simulink model "mrefrobotarm_modified_previous_y_previous_u_previous_ref_prepro"  (R2018b)
settings: Solver=FixedStepAuto  StartTime=0.0  StopTime=10  RelTol=1e-3  AbsTol=1e-6
undefined symbols (not defined in the file or in its folder): cc, options
libraries: neural x594, simulink x1
(part 4 of 22)

== system mrefrobotarm_modified_previous_y_previous_u_previous_ref_prepro/pre_0.01/Layer 3 ==
  "a{2} " : Inport  PortDimensions=30
      mask Display: e = 0.06;c1 = [120 230 180]/255;c2 = ([120 230 180]+0)/(256+128);c3 = ([120 230 180]+128)/(256+128);patch([0 1 1 0],[0 0 1 1],c1);patch([0 1 1 1-e 1-e 0+e],[0 0 1 1-e 0+e 0+e],c2);patch([0 0 1 1-e 0+e 0+e],[0 1 1 1-e 1-e 0+e],c3);plot([0 1 1 0 0],[0 0 1 1 0]);
  Delays 1 : Subsystem
      mask Display: e = 0.06;c1 = [120 150 230]/255;c2 = ([120 150 230]+0)/383;c3 = ([120 150 230]+128)/383;patch([0 1 1 0],[0 0 1 1],c1);patch([0 1 1 1-e 1-e 0+e],[0 0 1 1-e 0+e 0+e],c2);patch([0 0 1 1-e 0+e 0+e],[0 1 1 1-e 1-e 0+e],c3);plot([0 1 1 0 0],[0 0 1 1 0]);disp('0');
  "LW{3,2}" : Subsystem
      mask Display: e = 0.06;c1 = [120 150 230]/255;c2 = ([120 150 230]+0)/383;c3 = ([120 150 230]+128)/383;patch([0 1 1 0],[0 0 1 1],c1);patch([0 1 1 1-e 1-e 0+e],[0 0 1 1-e 0+e 0+e],c2);patch([0 0 1 1-e 0+e 0+e],[0 1 1 1-e 1-e 0+e],c3);plot([0 1 1 0 0],[0 0 1 1 0]);disp('W');
  "b{3}" : Constant  Value=0.10618203195990393028491638460764079354703426361083984375
      mask Display: e = 0.06;c1 = [120 150 230]/255;c2 = ([120 150 230]+0)/383;c3 = ([120 150 230]+128)/383;patch([0 1 1 0],[0 0 1 1],c1);patch([0 1 1 1-e 1-e 0+e],[0 0 1 1-e 0+e 0+e],c2);patch([0 0 1 1-e 0+e 0+e],[0 1 1 1-e 1-e 0+e],c3);plot([0 1 1 0 0],[0 0 1 1 0]);disp('b');
  netsum : Sum  Inputs=2  SaturateOnIntegerOverflow=on  InputSameDT=on  OutDataTypeStr=Inherit: Same as first input
      mask Display: e = 0.06;c1 = [120 150 230]/255;c2 = ([120 150 230]+0)/383;c3 = ([120 150 230]+128)/383;patch([0 1 1 0],[0 0 1 1],c1);patch([0 1 1 1-e 1-e 0+e],[0 0 1 1-e 0+e 0+e],c2);patch([0 0 1 1-e 0+e 0+e],[0 1 1 1-e 1-e 0+e],c3);plot([0 1 1 0 0],[0 0 1 1 0]);disp('+');
  purelin : neural/Transfer Functions/purelin
  "a{3}" : Outport  InitialOutput=0
      mask Display: e = 0.06;c1 = [120 230 180]/255;c2 = ([120 230 180]+0)/(256+128);c3 = ([120 230 180]+128)/(256+128);patch([0 1 1 0],[0 0 1 1],c1);patch([0 1 1 1-e 1-e 0+e],[0 0 1 1-e 0+e 0+e],c2);patch([0 0 1 1-e 0+e 0+e],[0 1 1 1-e 1-e 0+e],c3);plot([0 1 1 0 0],[0 0 1 1 0]);
  wires:
  "a{2} "/1 -> Delays 1/1("p{3}")
  Delays 1/1("pd{3,2}") -> "LW{3,2}"/1("ad{3,2}")
  "LW{3,2}"/1("lz{3,2}") -> netsum/1
  "b{3}"/1 -> netsum/2
  netsum/1 -> purelin/1
  purelin/1 -> "a{3}"/1

== system mrefrobotarm_modified_previous_y_previous_u_previous_ref_prepro/pre_0.01/Process Input 1 ==
  x : Inport  PortDimensions=10
      mask Display: e = 0.06;c1 = [120 230 180]/255;c2 = ([120 230 180]+0)/(256+128);c3 = ([120 230 180]+128)/(256+128);patch([0 1 1 0],[0 0 1 1],c1);patch([0 1 1 1-e 1-e 0+e],[0 0 1 1-e 0+e 0+e],c2);patch([0 0 1 1-e 0+e 0+e],[0 1 1 1-e 1-e 0+e],c3);plot([0 1 1 0 0],[0 0 1 1 0]);
  mapminmax : neural/Processing Functions/mapminmax  xmin=[-0.499622681643638155701836467415;-0.499622681643638155701836467415;-0.499622681643638155701836467415;-0.499622681643638155701836467415;-0.521390823259639368814077897696;-0.521390823259639368814077897696;-0.521390823259639368814077897696;-0.521390823259639368814077897696;-181.831597500088662400230532512;-181.831597500088662400230532512]  xmax=[0.499081940855403360934872125654;0.499081940855403360934872125654;0.499081940855403360934872125654;0.499081940855403360934872125654;0.529053256590264919800858933741;0.529053256590264919800858933741;0.529053256590264919800858933741;0.529053256590264919800858933741;187.244110317709044011280639097;187.244110317709044011280639097]  ymin=-1  ymax=1
  p : Outport  PortDimensions=10
      mask Display: e = 0.06;c1 = [120 230 180]/255;c2 = ([120 230 180]+0)/(256+128);c3 = ([120 230 180]+128)/(256+128);patch([0 1 1 0],[0 0 1 1],c1);patch([0 1 1 1-e 1-e 0+e],[0 0 1 1-e 0+e 0+e],c2);patch([0 0 1 1-e 0+e 0+e],[0 1 1 1-e 1-e 0+e],c3);plot([0 1 1 0 0],[0 0 1 1 0]);
  wires:
  x/1 -> mapminmax/1
  mapminmax/1 -> p/1

== system mrefrobotarm_modified_previous_y_previous_u_previous_ref_prepro/pre_0.01/Process Output 1 ==
  a : Inport  PortDimensions=1
      mask Display: e = 0.06;c1 = [120 230 180]/255;c2 = ([120 230 180]+0)/(256+128);c3 = ([120 230 180]+128)/(256+128);patch([0 1 1 0],[0 0 1 1],c1);patch([0 1 1 1-e 1-e 0+e],[0 0 1 1-e 0+e 0+e],c2);patch([0 0 1 1-e 0+e 0+e],[0 1 1 1-e 1-e 0+e],c3);plot([0 1 1 0 0],[0 0 1 1 0]);
  mapminmax_reverse : neural/Processing Functions/mapminmax_reverse  xmin=-181.831597500088662400230532512  xmax=187.244110317709044011280639097  ymin=-1  ymax=1
  y : Outport  PortDimensions=1
      mask Display: e = 0.06;c1 = [120 230 180]/255;c2 = ([120 230 180]+0)/(256+128);c3 = ([120 230 180]+128)/(256+128);patch([0 1 1 0],[0 0 1 1],c1);patch([0 1 1 1-e 1-e 0+e],[0 0 1 1-e 0+e 0+e],c2);patch([0 0 1 1-e 0+e 0+e],[0 1 1 1-e 1-e 0+e],c3);plot([0 1 1 0 0],[0 0 1 1 0]);
  wires:
  a/1 -> mapminmax_reverse/1
  mapminmax_reverse/1 -> y/1

== system mrefrobotarm_modified_previous_y_previous_u_previous_ref_prepro/m=0.01 sd =0.01/Layer 1/Delays 1 ==
  "p{1}" : Inport  PortDimensions=10
      mask Display: e = 0.06;c1 = [120 230 180]/255;c2 = ([120 230 180]+0)/(256+128);c3 = ([120 230 180]+128)/(256+128);patch([0 1 1 0],[0 0 1 1],c1);patch([0 1 1 1-e 1-e 0+e],[0 0 1 1-e 0+e 0+e],c2);patch([0 0 1 1-e 0+e 0+e],[0 1 1 1-e 1-e 0+e],c3);plot([0 1 1 0 0],[0 0 1 1 0]);
  mux : Mux  Inputs=1
      mask Display: e = 0.06;c1 = [120 150 230]/255;c2 = ([120 150 230]+0)/383;c3 = ([120 150 230]+128)/383;patch([0 1 1 0],[0 0 1 1],c1);patch([0 1 1 1-e 1-e 0+e],[0 0 1 1-e 0+e 0+e],c2);patch([0 0 1 1-e 0+e 0+e],[0 1 1 1-e 1-e 0+e],c3);plot([0 1 1 0 0],[0 0 1 1 0]);disp('Mux')
  "pd{1,1}" : Outport
      mask Display: e = 0.06;c1 = [120 230 180]/255;c2 = ([120 230 180]+0)/(256+128);c3 = ([120 230 180]+128)/(256+128);patch([0 1 1 0],[0 0 1 1],c1);patch([0 1 1 1-e 1-e 0+e],[0 0 1 1-e 0+e 0+e],c2);patch([0 0 1 1-e 0+e 0+e],[0 1 1 1-e 1-e 0+e],c3);plot([0 1 1 0 0],[0 0 1 1 0]);
  wires:
  "p{1}"/1 -> mux/1
  mux/1 -> "pd{1,1}"/1

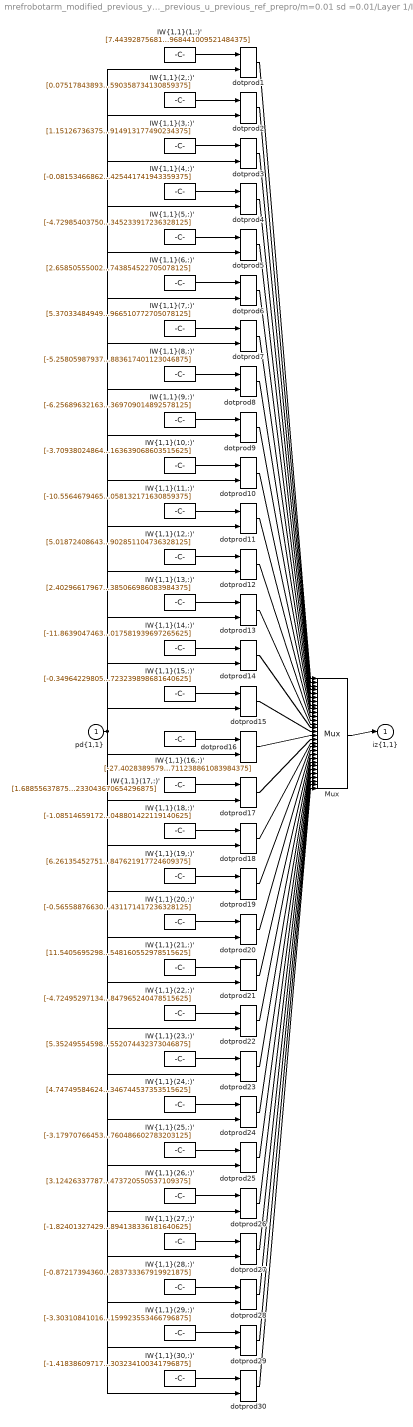
== system mrefrobotarm_modified_previous_y_previous_u_previous_ref_prepro/m=0.01 sd =0.01/Layer 1/IW{1,1} ==
  "pd{1,1}" : Inport  PortDimensions=10
      mask Display: e = 0.06;c1 = [120 230 180]/255;c2 = ([120 230 180]+0)/(256+128);c3 = ([120 230 180]+128)/(256+128);patch([0 1 1 0],[0 0 1 1],c1);patch([0 1 1 1-e 1-e 0+e],[0 0 1 1-e 0+e 0+e],c2);patch([0 0 1 1-e 0+e 0+e],[0 1 1 1-e 1-e 0+e],c3);plot([0 1 1 0 0],[0 0 1 1 0]);
  "IW{1,1}(1,:)'" : Constant  Value=[7.44392875681690302513970891595818102359771728515625;-4.6736656727683101308912227977998554706573486328125;-4.6390972498699891701789965736679732799530029296875;3.336024804118176145806273780181072652339935302734375;-0.105740361348570510724442783612175844609737396240234375;-3.024615511833397274443768765195272862911224365234375;2.36822163920083728072540907305665314197540283203125;-1.0457591878507825899902172750444151461124420166015625;1.046465722409650300761541075189597904682159423828125;-1.08392310721119056182715212344191968441009521484375]
      mask Display: e = 0.06;c1 = [120 150 230]/255;c2 = ([120 150 230]+0)/383;c3 = ([120 150 230]+128)/383;patch([0 1 1 0],[0 0 1 1],c1);patch([0 1 1 1-e 1-e 0+e],[0 0 1 1-e 0+e 0+e],c2);patch([0 0 1 1-e 0+e 0+e],[0 1 1 1-e 1-e 0+e],c3);plot([0 1 1 0 0],[0 0 1 1 0]);disp('Weights');
  "IW{1,1}(10,:)'" : Constant  Value=[-3.70938024864611026742977628600783646106719970703125;7.378455816069614314756108797155320644378662109375;-1.23455737014168942522474026191048324108123779296875;-0.80686346190143953815976374244200997054576873779296875;-2.678462781440510642738672686391510069370269775390625;-0.64571835168026459061962896157638169825077056884765625;0.99308648301582724826630510506220161914825439453125;0.0755819949909401211929349528872990049421787261962890625;-1.49364463106134603975760910543613135814666748046875;-1.0017750393580355794398428770364262163639068603515625]
      mask Display: e = 0.06;c1 = [120 150 230]/255;c2 = ([120 150 230]+0)/383;c3 = ([120 150 230]+128)/383;patch([0 1 1 0],[0 0 1 1],c1);patch([0 1 1 1-e 1-e 0+e],[0 0 1 1-e 0+e 0+e],c2);patch([0 0 1 1-e 0+e 0+e],[0 1 1 1-e 1-e 0+e],c3);plot([0 1 1 0 0],[0 0 1 1 0]);disp('Weights');
  "IW{1,1}(11,:)'" : Constant  Value=[-10.556467946534542790004707057960331439971923828125;5.98135936748858565437103607109747827053070068359375;3.653943008658041780023495448403991758823394775390625;-0.11845730388351143058667247487392160110175609588623046875;0.3526287060857471455932454773574136197566986083984375;1.7762225366593791253677636632346548140048980712890625;-1.37767047732931313674953344161622226238250732421875;-0.63824863500093720336536762260948307812213897705078125;0.8549609373443776139112060263869352638721466064453125;0.642023567932097360966281485161744058132171630859375]
      mask Display: e = 0.06;c1 = [120 150 230]/255;c2 = ([120 150 230]+0)/383;c3 = ([120 150 230]+128)/383;patch([0 1 1 0],[0 0 1 1],c1);patch([0 1 1 1-e 1-e 0+e],[0 0 1 1-e 0+e 0+e],c2);patch([0 0 1 1-e 0+e 0+e],[0 1 1 1-e 1-e 0+e],c3);plot([0 1 1 0 0],[0 0 1 1 0]);disp('Weights');
  "IW{1,1}(12,:)'" : Constant  Value=[5.018724086434847464488484547473490238189697265625;-4.47618638864089124496103977435268461704254150390625;1.4027950886756685999756655292003415524959564208984375;-0.01760069917661223615201748771141865290701389312744140625;0.06580408721141249583919119459096691571176052093505859375;-0.435612092762941827128742033892194740474224090576171875;-0.123377444074154851705316104926168918609619140625;1.513619026736596762106046298868022859096527099609375;-0.2081431014525624567657047236934886313974857330322265625;0.72520741288983459060801806117524392902851104736328125]
      mask Display: e = 0.06;c1 = [120 150 230]/255;c2 = ([120 150 230]+0)/383;c3 = ([120 150 230]+128)/383;patch([0 1 1 0],[0 0 1 1],c1);patch([0 1 1 1-e 1-e 0+e],[0 0 1 1-e 0+e 0+e],c2);patch([0 0 1 1-e 0+e 0+e],[0 1 1 1-e 1-e 0+e],c3);plot([0 1 1 0 0],[0 0 1 1 0]);disp('Weights');
  "IW{1,1}(13,:)'" : Constant  Value=[2.402966179675783298108626695466227829456329345703125;-1.6093946888288417351731141025084070861339569091796875;-0.0599342394857917681871839477025787346065044403076171875;-0.473275413721871374139738009034772403538227081298828125;-0.87682561446088513879004722184618003666400909423828125;0.22628827655378025429655508560244925320148468017578125;0.444344236189617103338633796738577075302600860595703125;-0.329101618948661689412205078042461536824703216552734375;-0.74224906653537059408876075394800864160060882568359375;-0.198310173910472453684405991225503385066986083984375]
      mask Display: e = 0.06;c1 = [120 150 230]/255;c2 = ([120 150 230]+0)/383;c3 = ([120 150 230]+128)/383;patch([0 1 1 0],[0 0 1 1],c1);patch([0 1 1 1-e 1-e 0+e],[0 0 1 1-e 0+e 0+e],c2);patch([0 0 1 1-e 0+e 0+e],[0 1 1 1-e 1-e 0+e],c3);plot([0 1 1 0 0],[0 0 1 1 0]);disp('Weights');
  "IW{1,1}(14,:)'" : Constant  Value=[-11.863904746364600129027166985906660556793212890625;12.5361553086397687906128339818678796291351318359375;-2.5443094142737994189928940613754093647003173828125;-0.01039113964185867967915388732080828049220144748687744140625;-1.4967394616593383549485452022054232656955718994140625;2.8221017636860725730230115004815161228179931640625;-0.1929962862818650481955273789935745298862457275390625;-2.793854429713266807056015750276856124401092529296875;-0.55739373934864355764062793241464532911777496337890625;-1.942644023618106619011314251110889017581939697265625]
      mask Display: e = 0.06;c1 = [120 150 230]/255;c2 = ([120 150 230]+0)/383;c3 = ([120 150 230]+128)/383;patch([0 1 1 0],[0 0 1 1],c1);patch([0 1 1 1-e 1-e 0+e],[0 0 1 1-e 0+e 0+e],c2);patch([0 0 1 1-e 0+e 0+e],[0 1 1 1-e 1-e 0+e],c3);plot([0 1 1 0 0],[0 0 1 1 0]);disp('Weights');
  "IW{1,1}(15,:)'" : Constant  Value=[-0.349642298058042089170527333408244885504245758056640625;2.606095277319749659028502719593234360218048095703125;-1.2963224095569134686201095973956398665904998779296875;-1.6246252820403725980469289424945600330829620361328125;4.39476319833291118044371614814735949039459228515625;0.327169101324004507613807390953297726809978485107421875;-3.431185950754114255545346168219111859798431396484375;0.82290277565416491967198453494347631931304931640625;1.922123395477147056453759432770311832427978515625;1.617192821484084053196284003206528723239898681640625]
      mask Display: e = 0.06;c1 = [120 150 230]/255;c2 = ([120 150 230]+0)/383;c3 = ([120 150 230]+128)/383;patch([0 1 1 0],[0 0 1 1],c1);patch([0 1 1 1-e 1-e 0+e],[0 0 1 1-e 0+e 0+e],c2);patch([0 0 1 1-e 0+e 0+e],[0 1 1 1-e 1-e 0+e],c3);plot([0 1 1 0 0],[0 0 1 1 0]);disp('Weights');
  "IW{1,1}(16,:)'" : Constant  Value=[-27.402838957925386154101943247951567173004150390625;27.31809732638254217818030156195163726806640625;4.187796846523848870447181980125606060028076171875;-0.58411520480238465768962896618177182972431182861328125;-2.421077128426197599964098117197863757610321044921875;-0.422057029001945249735427978521329350769519805908203125;0.46933164629719448246447655037627555429935455322265625;2.53884227966835052114902282482944428920745849609375;0.449642930046671496224774955408065579831600189208984375;-1.6588674943129804173480579265742562711238861083984375]
      mask Display: e = 0.06;c1 = [120 150 230]/255;c2 = ([120 150 230]+0)/383;c3 = ([120 150 230]+128)/383;patch([0 1 1 0],[0 0 1 1],c1);patch([0 1 1 1-e 1-e 0+e],[0 0 1 1-e 0+e 0+e],c2);patch([0 0 1 1-e 0+e 0+e],[0 1 1 1-e 1-e 0+e],c3);plot([0 1 1 0 0],[0 0 1 1 0]);disp('Weights');
  "IW{1,1}(17,:)'" : Constant  Value=[1.6885563787544148883768002633587457239627838134765625;-2.444624938858031004684789877501316368579864501953125;1.2252322902321706177275473237386904656887054443359375;-0.590265120460011782910214606090448796749114990234375;-0.332311297209722800172215784186846576631069183349609375;0.96575580482126255343899856598000042140483856201171875;-0.00354470077974646143037507073358938214369118213653564453125;-0.1126520435161915412169975070355576463043689727783203125;-0.33787689238072371455956499630701728165149688720703125;0.82478955221782601636704157499480061233043670654296875]
      mask Display: e = 0.06;c1 = [120 150 230]/255;c2 = ([120 150 230]+0)/383;c3 = ([120 150 230]+128)/383;patch([0 1 1 0],[0 0 1 1],c1);patch([0 1 1 1-e 1-e 0+e],[0 0 1 1-e 0+e 0+e],c2);patch([0 0 1 1-e 0+e 0+e],[0 1 1 1-e 1-e 0+e],c3);plot([0 1 1 0 0],[0 0 1 1 0]);disp('Weights');
  "IW{1,1}(18,:)'" : Constant  Value=[-1.0851465917204592415146180428564548492431640625;2.2300343259938220086269211606122553348541259765625;-0.275391438559908163785650003774208016693592071533203125;-0.3928571879931632704341382122947834432125091552734375;0.354493692437090335278782049499568529427051544189453125;-0.420219301105624498671176070274668745696544647216796875;-0.11256805056305159429275164484351989813148975372314453125;0.133925253068311878035245854334789328277111053466796875;-0.319742826625007747765039312071166932582855224609375;0.1931074981940363033405816395315923728048801422119140625]
      mask Display: e = 0.06;c1 = [120 150 230]/255;c2 = ([120 150 230]+0)/383;c3 = ([120 150 230]+128)/383;patch([0 1 1 0],[0 0 1 1],c1);patch([0 1 1 1-e 1-e 0+e],[0 0 1 1-e 0+e 0+e],c2);patch([0 0 1 1-e 0+e 0+e],[0 1 1 1-e 1-e 0+e],c3);plot([0 1 1 0 0],[0 0 1 1 0]);disp('Weights');
  "IW{1,1}(19,:)'" : Constant  Value=[6.2613545275196411665774576249532401561737060546875;-5.77393711359606864874649545527063310146331787109375;-0.44799036385010515548543708064244128763675689697265625;0.13038042920451109463186867287731729447841644287109375;-1.1128052994417583221320455777458846569061279296875;-0.68497464755320169871311009046621620655059814453125;1.488082305967609375585425368626601994037628173828125;-0.58498852802415501894728322440641932189464569091796875;-0.72696347840742070456343526529963128268718719482421875;-0.91570155227344718351645269649452529847621917724609375]
      mask Display: e = 0.06;c1 = [120 150 230]/255;c2 = ([120 150 230]+0)/383;c3 = ([120 150 230]+128)/383;patch([0 1 1 0],[0 0 1 1],c1);patch([0 1 1 1-e 1-e 0+e],[0 0 1 1-e 0+e 0+e],c2);patch([0 0 1 1-e 0+e 0+e],[0 1 1 1-e 1-e 0+e],c3);plot([0 1 1 0 0],[0 0 1 1 0]);disp('Weights');
  "IW{1,1}(2,:)'" : Constant  Value=[0.07517843893693586243553994563626474700868129730224609375;3.111042594677205119779728192952461540699005126953125;-2.72719944514824863546209599007852375507354736328125;-2.374128996332302232730171454022638499736785888671875;-0.484291377306462267338105220915167592465877532958984375;2.297251782196087166454390171566046774387359619140625;-1.9655189022791590414129814234911464154720306396484375;0.09551081790576276819848544619162566959857940673828125;1.7919979861660990660965353526989929378032684326171875;2.88238796171572797533144694170914590358734130859375]
      mask Display: e = 0.06;c1 = [120 150 230]/255;c2 = ([120 150 230]+0)/383;c3 = ([120 150 230]+128)/383;patch([0 1 1 0],[0 0 1 1],c1);patch([0 1 1 1-e 1-e 0+e],[0 0 1 1-e 0+e 0+e],c2);patch([0 0 1 1-e 0+e 0+e],[0 1 1 1-e 1-e 0+e],c3);plot([0 1 1 0 0],[0 0 1 1 0]);disp('Weights');
  "IW{1,1}(20,:)'" : Constant  Value=[-0.5655887663078853488940467286738567054271697998046875;0.653903601104851350811486554448492825031280517578125;-1.34929695276203975851103677996434271335601806640625;-0.356569327289411985848488484407425858080387115478515625;-2.467035815630168382739384469459764659404754638671875;4.1073377036829601394174460438080132007598876953125;-1.7883809654680782319502441168879158794879913330078125;0.146222307088537395447502831302699632942676544189453125;0.378437219084869713725538531434722244739532470703125;0.66357811677403788497286996062030084431171417236328125]
      mask Display: e = 0.06;c1 = [120 150 230]/255;c2 = ([120 150 230]+0)/383;c3 = ([120 150 230]+128)/383;patch([0 1 1 0],[0 0 1 1],c1);patch([0 1 1 1-e 1-e 0+e],[0 0 1 1-e 0+e 0+e],c2);patch([0 0 1 1-e 0+e 0+e],[0 1 1 1-e 1-e 0+e],c3);plot([0 1 1 0 0],[0 0 1 1 0]);disp('Weights');
  "IW{1,1}(21,:)'" : Constant  Value=[11.5405695298654169533847380080260336399078369140625;-12.65940146157516466018932987935841083526611328125;-1.4837236029238980439259876220603473484516143798828125;0.5934825145506030796838103924528695642948150634765625;2.6087113327163162779243066324852406978607177734375;-0.99095465263819015877544416071032173931598663330078125;-0.586222874234343382937595379189588129520416259765625;1.649770440132100279839733047992922365665435791015625;2.600883961520991771720900942455045878887176513671875;1.2459563927813219752493978376151062548160552978515625]
      mask Display: e = 0.06;c1 = [120 150 230]/255;c2 = ([120 150 230]+0)/383;c3 = ([120 150 230]+128)/383;patch([0 1 1 0],[0 0 1 1],c1);patch([0 1 1 1-e 1-e 0+e],[0 0 1 1-e 0+e 0+e],c2);patch([0 0 1 1-e 0+e 0+e],[0 1 1 1-e 1-e 0+e],c3);plot([0 1 1 0 0],[0 0 1 1 0]);disp('Weights');
  "IW{1,1}(22,:)'" : Constant  Value=[-4.72495297134443870135100951301865279674530029296875;-3.6612758066156505520893915672786533832550048828125;9.1307356427337378335096218506805598735809326171875;-1.6514122347745334717927789824898354709148406982421875;-0.94481991805823162255961733535514213144779205322265625;3.389752710337073704494059711578302085399627685546875;-2.691142831870891871659523530979640781879425048828125;-1.5547670892227956063180727142025716602802276611328125;0.6594750666437523278773369383998215198516845703125;0.2308273689137200490595347446287632919847965240478515625]
      mask Display: e = 0.06;c1 = [120 150 230]/255;c2 = ([120 150 230]+0)/383;c3 = ([120 150 230]+128)/383;patch([0 1 1 0],[0 0 1 1],c1);patch([0 1 1 1-e 1-e 0+e],[0 0 1 1-e 0+e 0+e],c2);patch([0 0 1 1-e 0+e 0+e],[0 1 1 1-e 1-e 0+e],c3);plot([0 1 1 0 0],[0 0 1 1 0]);disp('Weights');
  "IW{1,1}(23,:)'" : Constant  Value=[5.35249554598566934515702087082900106906890869140625;-8.3947052042032481722344527952373027801513671875;5.20674656749528974586382901179604232311248779296875;0.1057961470926972735728810448563308455049991607666015625;0.484913147426727253463951683443156071007251739501953125;0.304219401861873184333973085813340730965137481689453125;-1.225153512517460629993593101971782743930816650390625;0.6788050534317513484694472936098463833332061767578125;-1.1973619723788748725468167322105728089809417724609375;-0.1013175564166879094596396271299454383552074432373046875]
      mask Display: e = 0.06;c1 = [120 150 230]/255;c2 = ([120 150 230]+0)/383;c3 = ([120 150 230]+128)/383;patch([0 1 1 0],[0 0 1 1],c1);patch([0 1 1 1-e 1-e 0+e],[0 0 1 1-e 0+e 0+e],c2);patch([0 0 1 1-e 0+e 0+e],[0 1 1 1-e 1-e 0+e],c3);plot([0 1 1 0 0],[0 0 1 1 0]);disp('Weights');
  "IW{1,1}(24,:)'" : Constant  Value=[4.7474958462455081331654582754708826541900634765625;-0.56139374161379773653379743336699903011322021484375;-2.551788953760051992247781527112238109111785888671875;-0.99778767395680867391405399757786653935909271240234375;-0.34030095527620451978378923740820027887821197509765625;-1.27599383979261293831086732097901403903961181640625;1.186934513853181716314111326937563717365264892578125;0.8604641122355964899526270528440363705158233642578125;-0.153556002938787461431502379127778112888336181640625;-0.12256042654575038941544562476337887346744537353515625]
      mask Display: e = 0.06;c1 = [120 150 230]/255;c2 = ([120 150 230]+0)/383;c3 = ([120 150 230]+128)/383;patch([0 1 1 0],[0 0 1 1],c1);patch([0 1 1 1-e 1-e 0+e],[0 0 1 1-e 0+e 0+e],c2);patch([0 0 1 1-e 0+e 0+e],[0 1 1 1-e 1-e 0+e],c3);plot([0 1 1 0 0],[0 0 1 1 0]);disp('Weights');
  "IW{1,1}(25,:)'" : Constant  Value=[-3.1797076645325699217892179149203002452850341796875;3.734294835475939322577687562443315982818603515625;1.86538514582187797685719488072209060192108154296875;-3.577523184763872432512243904056958854198455810546875;-0.1801846616331347072925694874356850050389766693115234375;0.842643107149921188891994461300782859325408935546875;-0.7368706843575132392487603283370845019817352294921875;-1.1996527136506200950094580548466183245182037353515625;-0.346079193916736194136518633968080393970012664794921875;-0.396694308283962737693428834973019547760486602783203125]
      mask Display: e = 0.06;c1 = [120 150 230]/255;c2 = ([120 150 230]+0)/383;c3 = ([120 150 230]+128)/383;patch([0 1 1 0],[0 0 1 1],c1);patch([0 1 1 1-e 1-e 0+e],[0 0 1 1-e 0+e 0+e],c2);patch([0 0 1 1-e 0+e 0+e],[0 1 1 1-e 1-e 0+e],c3);plot([0 1 1 0 0],[0 0 1 1 0]);disp('Weights');
  "IW{1,1}(26,:)'" : Constant  Value=[3.12426337787707897319933181279338896274566650390625;-4.36624704298784305223080082214437425136566162109375;3.2575199274810824334736025775782763957977294921875;-3.431769755768558471942242249497212469577789306640625;-0.054498989908941510018625109523782157339155673980712890625;0.36689560986312896861960552996606566011905670166015625;0.6856860813167833246239979416714049875736236572265625;1.6297863103363916525978538629715330898761749267578125;1.3371353193966777350709662641747854650020599365234375;1.093416193759926269279958432889543473720550537109375]
      mask Display: e = 0.06;c1 = [120 150 230]/255;c2 = ([120 150 230]+0)/383;c3 = ([120 150 230]+128)/383;patch([0 1 1 0],[0 0 1 1],c1);patch([0 1 1 1-e 1-e 0+e],[0 0 1 1-e 0+e 0+e],c2);patch([0 0 1 1-e 0+e 0+e],[0 1 1 1-e 1-e 0+e],c3);plot([0 1 1 0 0],[0 0 1 1 0]);disp('Weights');
  "IW{1,1}(27,:)'" : Constant  Value=[-1.8240132742958525824406024185009300708770751953125;3.665467649823689999522002835874445736408233642578125;-0.08099650826464015185290890030955779366195201873779296875;-0.57947593984516121423666845657862722873687744140625;1.1343794714281141278178210995974950492382049560546875;-1.1901217688666794192187126100179739296436309814453125;-0.66956421189875914290468017497914843261241912841796875;1.6359404457898414353422822387074120342731475830078125;0.1925093816509529653924204239956452511250972747802734375;0.2239375878662033247934459723182953894138336181640625]
      mask Display: e = 0.06;c1 = [120 150 230]/255;c2 = ([120 150 230]+0)/383;c3 = ([120 150 230]+128)/383;patch([0 1 1 0],[0 0 1 1],c1);patch([0 1 1 1-e 1-e 0+e],[0 0 1 1-e 0+e 0+e],c2);patch([0 0 1 1-e 0+e 0+e],[0 1 1 1-e 1-e 0+e],c3);plot([0 1 1 0 0],[0 0 1 1 0]);disp('Weights');
  "IW{1,1}(28,:)'" : Constant  Value=[-0.872173943607633450625371551723219454288482666015625;5.25512164419217153721319846226833760738372802734375;-4.685331785963711581644020043313503265380859375;0.834289299808426587645726613118313252925872802734375;-2.1762573927168897824913074146024882793426513671875;0.130140889257105596410468706380925141274929046630859375;2.129037893274777548668907911633141338825225830078125;-0.88145543343128374136341562916641123592853546142578125;-1.4446731616323564839632354050991125404834747314453125;-1.7558968253077729126943040682817809283733367919921875]
      mask Display: e = 0.06;c1 = [120 150 230]/255;c2 = ([120 150 230]+0)/383;c3 = ([120 150 230]+128)/383;patch([0 1 1 0],[0 0 1 1],c1);patch([0 1 1 1-e 1-e 0+e],[0 0 1 1-e 0+e 0+e],c2);patch([0 0 1 1-e 0+e 0+e],[0 1 1 1-e 1-e 0+e],c3);plot([0 1 1 0 0],[0 0 1 1 0]);disp('Weights');
  "IW{1,1}(29,:)'" : Constant  Value=[-3.30310841016261402813825043267570436000823974609375;-4.65377868158993290848002288839779794216156005859375;1.75878706131269613166523413383401930332183837890625;4.69135890776618680320098064839839935302734375;-3.467606116087420087268355928245000541210174560546875;0.56924689976836539972993023184244520962238311767578125;3.264673395387816423607318938593380153179168701171875;-3.494399385547103609184205197379924356937408447265625;-0.59184052372902884453509386730729602277278900146484375;0.54438173488576768743740785794216208159923553466796875]
      mask Display: e = 0.06;c1 = [120 150 230]/255;c2 = ([120 150 230]+0)/383;c3 = ([120 150 230]+128)/383;patch([0 1 1 0],[0 0 1 1],c1);patch([0 1 1 1-e 1-e 0+e],[0 0 1 1-e 0+e 0+e],c2);patch([0 0 1 1-e 0+e 0+e],[0 1 1 1-e 1-e 0+e],c3);plot([0 1 1 0 0],[0 0 1 1 0]);disp('Weights');
  "IW{1,1}(3,:)'" : Constant  Value=[1.1512673637556034567097640319843776524066925048828125;-5.53737976013809518605057746754027903079986572265625;2.564168777264312470975937685579992830753326416015625;0.19625559815241444550082405839930288493633270263671875;-0.485151448053758704848092975225881673395633697509765625;0.93104748155003125287265675069647841155529022216796875;-0.250923796589592795758250076687545515596866607666015625;-1.22774378303464093420416247681714594364166259765625;0.3874723104310648924553106553503312170505523681640625;-0.028228333698335515700161835184189840219914913177490234375]
      mask Display: e = 0.06;c1 = [120 150 230]/255;c2 = ([120 150 230]+0)/383;c3 = ([120 150 230]+128)/383;patch([0 1 1 0],[0 0 1 1],c1);patch([0 1 1 1-e 1-e 0+e],[0 0 1 1-e 0+e 0+e],c2);patch([0 0 1 1-e 0+e 0+e],[0 1 1 1-e 1-e 0+e],c3);plot([0 1 1 0 0],[0 0 1 1 0]);disp('Weights');
  "IW{1,1}(30,:)'" : Constant  Value=[-1.4183860971787429772206223788089118897914886474609375;-0.8170855934133374187666731813806109130382537841796875;4.7571480098223464239026725408621132373809814453125;-4.11771715428997442387526461970992386341094970703125;-1.1259252277220845872562904332880862057209014892578125;0.8885099481654552544540592862176708877086639404296875;1.2843821574967917431564501384855248034000396728515625;-2.059691264050130588003639786620624363422393798828125;-0.8720189695034203936074845842085778713226318359375;-0.95495030232230238009805134424823336303234100341796875]
      mask Display: e = 0.06;c1 = [120 150 230]/255;c2 = ([120 150 230]+0)/383;c3 = ([120 150 230]+128)/383;patch([0 1 1 0],[0 0 1 1],c1);patch([0 1 1 1-e 1-e 0+e],[0 0 1 1-e 0+e 0+e],c2);patch([0 0 1 1-e 0+e 0+e],[0 1 1 1-e 1-e 0+e],c3);plot([0 1 1 0 0],[0 0 1 1 0]);disp('Weights');
  "IW{1,1}(4,:)'" : Constant  Value=[-0.08153466862124426894897766260328353382647037506103515625;-0.68156154414485292658554271838511340320110321044921875;-0.7244008116259805785119851861963979899883270263671875;0.1628923928770475704208564593500341288745403289794921875;0.930012488062001541067047583055682480335235595703125;0.624584053000497352314823729102499783039093017578125;-0.416751672046266008475612352413008920848369598388671875;-0.78640669268823082393993217920069582760334014892578125;-0.12112611523055845375029804245059494860470294952392578125;0.4327741577922805671363448709598742425441741943359375]
      mask Display: e = 0.06;c1 = [120 150 230]/255;c2 = ([120 150 230]+0)/383;c3 = ([120 150 230]+128)/383;patch([0 1 1 0],[0 0 1 1],c1);patch([0 1 1 1-e 1-e 0+e],[0 0 1 1-e 0+e 0+e],c2);patch([0 0 1 1-e 0+e 0+e],[0 1 1 1-e 1-e 0+e],c3);plot([0 1 1 0 0],[0 0 1 1 0]);disp('Weights');
  "IW{1,1}(5,:)'" : Constant  Value=[-4.729854037502928321146100643090903759002685546875;10.6538218289730810539595040609128773212432861328125;-10.004828623033372281270203529857099056243896484375;5.9966033770067479480303518357686698436737060546875;-2.764430131988798056141831693821586668491363525390625;5.1835882880337056377584303845651447772979736328125;-0.2271440316044763818581486702896654605865478515625;-4.7546472048093217921405084780417382717132568359375;-3.4779913156446813360389569425024092197418212890625;-0.63613107628134912818751445229281671345233917236328125]
      mask Display: e = 0.06;c1 = [120 150 230]/255;c2 = ([120 150 230]+0)/383;c3 = ([120 150 230]+128)/383;patch([0 1 1 0],[0 0 1 1],c1);patch([0 1 1 1-e 1-e 0+e],[0 0 1 1-e 0+e 0+e],c2);patch([0 0 1 1-e 0+e 0+e],[0 1 1 1-e 1-e 0+e],c3);plot([0 1 1 0 0],[0 0 1 1 0]);disp('Weights');
  "IW{1,1}(6,:)'" : Constant  Value=[2.658505550025621833043487640679813921451568603515625;0.39067563978080210862486865153186954557895660400390625;-1.340300520228641545372738619334995746612548828125;-3.4817278062364334090261763776652514934539794921875;-3.786800075333292436852161699789576232433319091796875;7.38857135530607678219894296489655971527099609375;-6.85550852915829267431035987101495265960693359375;4.60341985404955078564626091974787414073944091796875;0.92167268789393330674641902078292332589626312255859375;0.069227546380084437060986601863987743854522705078125]
      mask Display: e = 0.06;c1 = [120 150 230]/255;c2 = ([120 150 230]+0)/383;c3 = ([120 150 230]+128)/383;patch([0 1 1 0],[0 0 1 1],c1);patch([0 1 1 1-e 1-e 0+e],[0 0 1 1-e 0+e 0+e],c2);patch([0 0 1 1-e 0+e 0+e],[0 1 1 1-e 1-e 0+e],c3);plot([0 1 1 0 0],[0 0 1 1 0]);disp('Weights');
  "IW{1,1}(7,:)'" : Constant  Value=[5.37033484949713457723419196554459631443023681640625;2.48425644015792901342365439631976187229156494140625;-8.3234479175373987658304031356237828731536865234375;1.4730624561860417021108560220454819500446319580078125;-1.5401282611605033867618885778938420116901397705078125;-1.0681564838651713689188227363047190010547637939453125;1.0259359799327645301758593632257543504238128662109375;-0.1056761343645743200791997651322162710130214691162109375;-0.85170302891138394141279377436148934066295623779296875;-2.69184409165068405656029426609165966510772705078125]
      mask Display: e = 0.06;c1 = [120 150 230]/255;c2 = ([120 150 230]+0)/383;c3 = ([120 150 230]+128)/383;patch([0 1 1 0],[0 0 1 1],c1);patch([0 1 1 1-e 1-e 0+e],[0 0 1 1-e 0+e 0+e],c2);patch([0 0 1 1-e 0+e 0+e],[0 1 1 1-e 1-e 0+e],c3);plot([0 1 1 0 0],[0 0 1 1 0]);disp('Weights');
  "IW{1,1}(8,:)'" : Constant  Value=[-5.25805987937673879883959671133197844028472900390625;6.9557500281106161565958245773799717426300048828125;0.218611258015503795437695089276530779898166656494140625;0.32040413473526430099269646234461106359958648681640625;-0.62898519567057686874278488176059909164905548095703125;-1.070858822110146935102648058091290295124053955078125;1.2490790179807935711409072609967552125453948974609375;-0.9191240731767680305352996583678759634494781494140625;-0.92787657053103800297577663513948209583759307861328125;0.01195435596070441690297325720848675700835883617401123046875]
      mask Display: e = 0.06;c1 = [120 150 230]/255;c2 = ([120 150 230]+0)/383;c3 = ([120 150 230]+128)/383;patch([0 1 1 0],[0 0 1 1],c1);patch([0 1 1 1-e 1-e 0+e],[0 0 1 1-e 0+e 0+e],c2);patch([0 0 1 1-e 0+e 0+e],[0 1 1 1-e 1-e 0+e],c3);plot([0 1 1 0 0],[0 0 1 1 0]);disp('Weights');
  "IW{1,1}(9,:)'" : Constant  Value=[-6.25689632163533193676130395033396780490875244140625;5.77122284224883852488119373447261750698089599609375;0.44620835882717602149938329603173770010471343994140625;-0.129276999068928477587547831717529334127902984619140625;1.1097920050779535028340205826680175960063934326171875;0.68465956878291145404347162184421904385089874267578125;-1.48531967794987718178845170768909156322479248046875;0.5834898609339747022062283576815389096736907958984375;0.723607161065681570022434243583120405673980712890625;0.914602837597204398889516596682369709014892578125]
      mask Display: e = 0.06;c1 = [120 150 230]/255;c2 = ([120 150 230]+0)/383;c3 = ([120 150 230]+128)/383;patch([0 1 1 0],[0 0 1 1],c1);patch([0 1 1 1-e 1-e 0+e],[0 0 1 1-e 0+e 0+e],c2);patch([0 0 1 1-e 0+e 0+e],[0 1 1 1-e 1-e 0+e],c3);plot([0 1 1 0 0],[0 0 1 1 0]);disp('Weights');
  Mux : Mux  Inputs=30
      mask Display: e = 0.06;c1 = [120 150 230]/255;c2 = ([120 150 230]+0)/383;c3 = ([120 150 230]+128)/383;patch([0 1 1 0],[0 0 1 1],c1);patch([0 1 1 1-e 1-e 0+e],[0 0 1 1-e 0+e 0+e],c2);patch([0 0 1 1-e 0+e 0+e],[0 1 1 1-e 1-e 0+e],c3);plot([0 1 1 0 0],[0 0 1 1 0]);disp('Mux');
  dotprod{1..30} (30 alike) : neural/Weight Functions/dotprod
  "iz{1,1}" : Outport
      mask Display: e = 0.06;c1 = [120 230 180]/255;c2 = ([120 230 180]+0)/(256+128);c3 = ([120 230 180]+128)/(256+128);patch([0 1 1 0],[0 0 1 1],c1);patch([0 1 1 1-e 1-e 0+e],[0 0 1 1-e 0+e 0+e],c2);patch([0 0 1 1-e 0+e 0+e],[0 1 1 1-e 1-e 0+e],c3);plot([0 1 1 0 0],[0 0 1 1 0]);
  wires:
  "IW{1,1}(1,:)'"/1 -> dotprod1/1
  "pd{1,1}"/1 -> dotprod1/2, dotprod2/2, dotprod3/2, dotprod4/2, dotprod5/2, dotprod6/2, dotprod7/2, dotprod8/2, dotprod9/2, dotprod10/2, dotprod11/2, dotprod12/2, dotprod13/2, dotprod14/2, dotprod15/2, dotprod16/2, dotprod17/2, dotprod18/2, dotprod19/2, dotprod20/2, dotprod21/2, dotprod22/2, dotprod23/2, dotprod24/2, dotprod25/2, dotprod26/2, dotprod27/2, dotprod28/2, dotprod29/2, dotprod30/2
  dotprod1/1 -> Mux/1
  "IW{1,1}(2,:)'"/1 -> dotprod2/1
  dotprod2/1 -> Mux/2
  "IW{1,1}(3,:)'"/1 -> dotprod3/1
  dotprod3/1 -> Mux/3
  "IW{1,1}(4,:)'"/1 -> dotprod4/1
  dotprod4/1 -> Mux/4
  "IW{1,1}(5,:)'"/1 -> dotprod5/1
  dotprod5/1 -> Mux/5
  "IW{1,1}(6,:)'"/1 -> dotprod6/1
  dotprod6/1 -> Mux/6
  "IW{1,1}(7,:)'"/1 -> dotprod7/1
  dotprod7/1 -> Mux/7
  "IW{1,1}(8,:)'"/1 -> dotprod8/1
  dotprod8/1 -> Mux/8
  "IW{1,1}(9,:)'"/1 -> dotprod9/1
  dotprod9/1 -> Mux/9
  "IW{1,1}(10,:)'"/1 -> dotprod10/1
  dotprod10/1 -> Mux/10
  "IW{1,1}(11,:)'"/1 -> dotprod11/1
  dotprod11/1 -> Mux/11
  "IW{1,1}(12,:)'"/1 -> dotprod12/1
  dotprod12/1 -> Mux/12
  "IW{1,1}(13,:)'"/1 -> dotprod13/1
  dotprod13/1 -> Mux/13
  "IW{1,1}(14,:)'"/1 -> dotprod14/1
  dotprod14/1 -> Mux/14
  "IW{1,1}(15,:)'"/1 -> dotprod15/1
  dotprod15/1 -> Mux/15
  "IW{1,1}(16,:)'"/1 -> dotprod16/1
  dotprod16/1 -> Mux/16
  "IW{1,1}(17,:)'"/1 -> dotprod17/1
  dotprod17/1 -> Mux/17
  "IW{1,1}(18,:)'"/1 -> dotprod18/1
  dotprod18/1 -> Mux/18
  "IW{1,1}(19,:)'"/1 -> dotprod19/1
  dotprod19/1 -> Mux/19
  "IW{1,1}(20,:)'"/1 -> dotprod20/1
  dotprod20/1 -> Mux/20
  "IW{1,1}(21,:)'"/1 -> dotprod21/1
  dotprod21/1 -> Mux/21
  "IW{1,1}(22,:)'"/1 -> dotprod22/1
  dotprod22/1 -> Mux/22
  "IW{1,1}(23,:)'"/1 -> dotprod23/1
  dotprod23/1 -> Mux/23
  "IW{1,1}(24,:)'"/1 -> dotprod24/1
  dotprod24/1 -> Mux/24
  "IW{1,1}(25,:)'"/1 -> dotprod25/1
  dotprod25/1 -> Mux/25
  "IW{1,1}(26,:)'"/1 -> dotprod26/1
  dotprod26/1 -> Mux/26
  "IW{1,1}(27,:)'"/1 -> dotprod27/1
  dotprod27/1 -> Mux/27
  "IW{1,1}(28,:)'"/1 -> dotprod28/1
  dotprod28/1 -> Mux/28
  "IW{1,1}(29,:)'"/1 -> dotprod29/1
  dotprod29/1 -> Mux/29
  "IW{1,1}(30,:)'"/1 -> dotprod30/1
  dotprod30/1 -> Mux/30
  Mux/1 -> "iz{1,1}"/1

== system mrefrobotarm_modified_previous_y_previous_u_previous_ref_prepro/m=0.01 sd =0.01/Layer 2/Delays 1 ==
  "p{2}" : Inport  PortDimensions=30
      mask Display: e = 0.06;c1 = [120 230 180]/255;c2 = ([120 230 180]+0)/(256+128);c3 = ([120 230 180]+128)/(256+128);patch([0 1 1 0],[0 0 1 1],c1);patch([0 1 1 1-e 1-e 0+e],[0 0 1 1-e 0+e 0+e],c2);patch([0 0 1 1-e 0+e 0+e],[0 1 1 1-e 1-e 0+e],c3);plot([0 1 1 0 0],[0 0 1 1 0]);
  mux : Mux  Inputs=1
      mask Display: e = 0.06;c1 = [120 150 230]/255;c2 = ([120 150 230]+0)/383;c3 = ([120 150 230]+128)/383;patch([0 1 1 0],[0 0 1 1],c1);patch([0 1 1 1-e 1-e 0+e],[0 0 1 1-e 0+e 0+e],c2);patch([0 0 1 1-e 0+e 0+e],[0 1 1 1-e 1-e 0+e],c3);plot([0 1 1 0 0],[0 0 1 1 0]);disp('Mux')
  "pd{2,1}" : Outport
      mask Display: e = 0.06;c1 = [120 230 180]/255;c2 = ([120 230 180]+0)/(256+128);c3 = ([120 230 180]+128)/(256+128);patch([0 1 1 0],[0 0 1 1],c1);patch([0 1 1 1-e 1-e 0+e],[0 0 1 1-e 0+e 0+e],c2);patch([0 0 1 1-e 0+e 0+e],[0 1 1 1-e 1-e 0+e],c3);plot([0 1 1 0 0],[0 0 1 1 0]);
  wires:
  "p{2}"/1 -> mux/1
  mux/1 -> "pd{2,1}"/1
